simulink model "Differntial_Equation7DOF"  (R2022b)
settings: Solver=ode1  StartTime=0.0  StopTime=50  FixedStep=1e-3  RelTol=1e-3
values from neighbouring files (symbols this model uses):
  cxyz = zeros(1,21)    [Simulation_7DOF.m]
  inertia_i = [0.1,0,0,0,0.09,0,0,0,0.02,0.05,0,0,0,0.018,0,0,0,0.044,0.08,0,0,0,0.075,0,0,0,0.01,0.03,0,0,0,0.01,0,0,0,0.029,0.02,0,0,0,0.018,0,0,0,0.05,0.005,0,0,0,0.0036,0,0,0,0.0047,0.001,0,0,0,0.001,0,0,0,0.001]'    [Simulation_7DOF.m]
  initial_condition_q7 = [0,0,0,0,0,0,0]    [Simulation_7DOF.m]
settings Model: Creator=djama  LastModifiedBy=djama

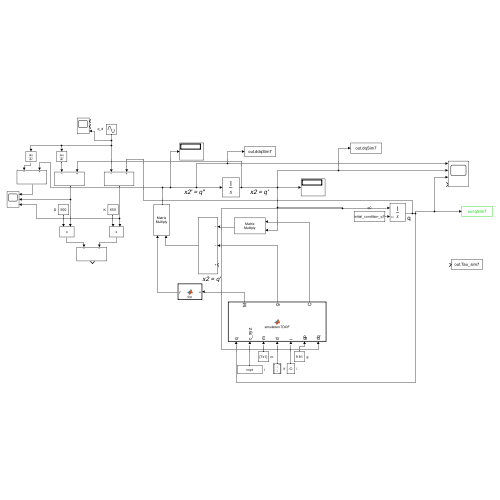
[thumbnail: Simulink's stored preview of the top-level diagram]
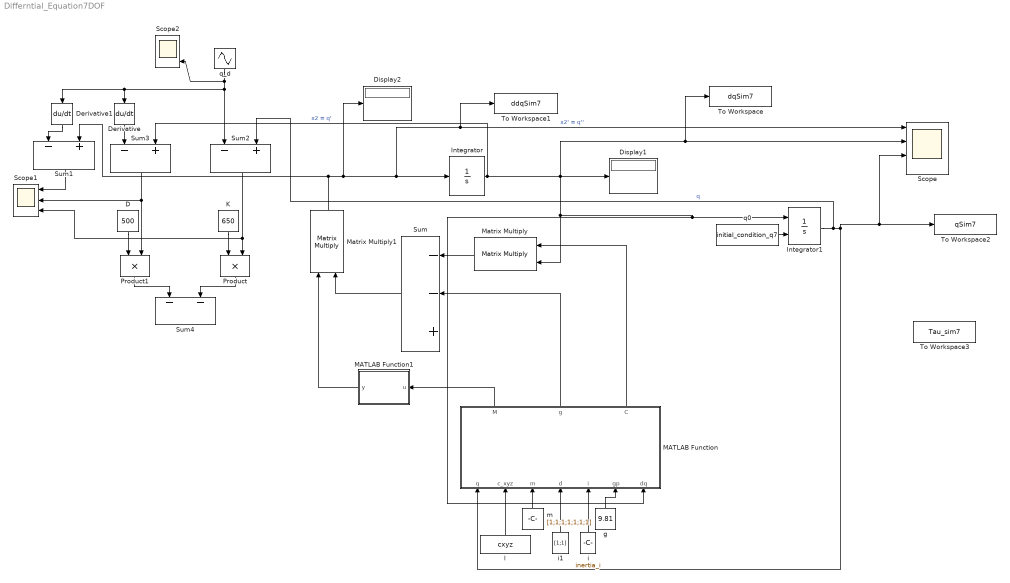
== system Differntial_Equation7DOF ==
  D : Constant  Value=500
  Derivative : Derivative
  Derivative1 : Derivative
  Display1 : Display
  Display2 : Display
  Integrator : Integrator  InitialCondition=[0.1;0.1;0;0;0;0;0]
  Integrator1 : Integrator  InitialConditionSource=external  InitialCondition=[pi/2;-pi/4]
  K : Constant  Value=650
  MATLAB Function : MATLAB Function  TreatAsAtomicUnit=on
  MATLAB Function1 : MATLAB Function  TreatAsAtomicUnit=on
  Matrix Multiply : Product  Multiplication=Matrix(*)
  Matrix Multiply1 : Product  Multiplication=Matrix(*)
  Product : Product
  Product1 : Product
  Scope : Scope  NumInputPorts=4
  Scope1 : Scope  NumInputPorts=3
  Scope2 : Scope  NumInputPorts=3
  Sum : Sum  Inputs=--+
  Sum1 : Sum  Inputs=-+
  Sum2 : Sum  Inputs=-+
  Sum3 : Sum  Inputs=-+
  Sum4 : Sum  Inputs=--
  To Workspace : ToWorkspace  VariableName=dqSim7  SaveFormat=Timeseries  SampleTime=0.1
  To Workspace1 : ToWorkspace  VariableName=ddqSim7  SaveFormat=Timeseries  SampleTime=0.1
  To Workspace2 : ToWorkspace  VariableName=qSim7  SaveFormat=Timeseries  SampleTime=0.1
  To Workspace3 : ToWorkspace  VariableName=Tau_sim7  SaveFormat=Timeseries  SampleTime=0.1
  g : Constant  Value=9.81
  i : Constant  Value=inertia_i  VectorParams1D=off
  i1 : Constant  Value=[1;1]  VectorParams1D=off
  l : Constant  Value=cxyz  VectorParams1D=off
  m : Constant  Value=[1;1;1;1;1;1;1]  VectorParams1D=off
  q0 : Constant  Value=initial_condition_q7
  "q_d " : Sin  Amplitude=[0.1,0.1,0.1,0.1,0.1,0.1,0.1]*10  SampleTime=0
  wires:
  Integrator/1 -> Sum3/2, To Workspace/1, Scope/2, Matrix Multiply/2, MATLAB Function/7(dq), Integrator1/1, Display1/1  "x2 = q'"
  Sum/1 -> Matrix Multiply1/2
  Sum3/1 -> Product1/2, Scope1/2
  q0/1 -> Integrator1/2
  Sum2/1 -> Scope1/3, Product/2
  g/1 -> MATLAB Function/6(gp)
  Integrator1/1 -> Sum2/2, Scope/3, To Workspace2/1, MATLAB Function/1(q)  "q"
  Product1/1 -> Sum4/1
  Matrix Multiply/1 -> Sum/1
  D/1 -> Product1/1
  i/1 -> MATLAB Function/5(i)
  MATLAB Function1/1(y) -> Matrix Multiply1/1
  MATLAB Function/2(g) -> Sum/2
  Derivative/1 -> Sum3/1
  MATLAB Function/3(C) -> Matrix Multiply/1
  Matrix Multiply1/1 -> To Workspace1/1, Scope/1, Integrator/1, Display2/1, Sum1/2  "x2' = q''"
  MATLAB Function/1(M) -> MATLAB Function1/1(u)
  m/1 -> MATLAB Function/3(m)
  K/1 -> Product/1
  l/1 -> MATLAB Function/2(c_xyz)
  Product/1 -> Sum4/2
  i1/1 -> MATLAB Function/4(d)
  Derivative1/1 -> Sum1/1
  Sum1/1 -> Scope1/1
  "q_d "/1 -> Scope2/3, Derivative1/1, Derivative/1, Sum2/1

== matlab function Differntial_Equation7DOF/MATLAB Function1 ==
  data: u input; y output
function y = fcn(u)

y = inv(u);

== matlab function Differntial_Equation7DOF/MATLAB Function ==
  data: q input; c_xyz input; m input; d input; i input; gp input; M output; g output; C output; dq input
function [M,g,C] = simulation7DOF(q,c_xyz,m,d,i,gp,dq)
%Befüllen der Matrizen mit den Beispielwerten
M = M_kukalwr_nom(m,c_xyz,d,i,q); 
C = C_kukalwr_nom(m,c_xyz,d,i,q,dq);
g = g_kukalwr_nom(gp,m,c_xyz,d,q); 
end
